simulink model "pitch_loop"  (Simulink 8.2)
settings: Solver=ode45  StartTime=0.0  StopTime=500  FixedStep=0.01  RelTol=1e-3
undefined symbols (not defined in the file): P
settings Model: Creator=paul  LastModifiedBy=paul
settings DataIOCC: SignalLoggingSaveFormat=Dataset
settings OptimizationCC: ExpressionDepthLimit=128
settings DebuggingCC: FcnCallInpInsideContextMsg=EnableAllAsError  StateNameClashWarn=none
settings GRTTargetCC: CombineOutputUpdateFcns=on  GRTInterface=off

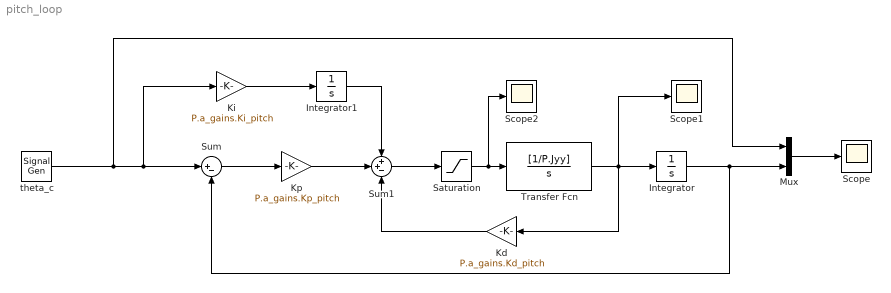
== system pitch_loop ==
  Integrator : Integrator
  Integrator1 : Integrator
  Kd : Gain  Gain=P.a_gains.Kd_pitch
  Ki : Gain  Gain=P.a_gains.Ki_pitch
  Kp : Gain  Gain=P.a_gains.Kp_pitch
  Mux : Mux  Inputs=2
  Saturation : Saturate  UpperLimit=P.T_theta_max  LowerLimit=-P.T_theta_max
  Scope : Scope
  Scope1 : Scope
  Scope2 : Scope
      settings: SaveName=ScopeData2
  Sum : Sum  Inputs=|+-
  Sum1 : Sum  Inputs=++-
  Transfer Fcn : TransferFcn  Numerator=[1/P.Jyy]  Denominator=[1 0]
  theta_c : SignalGenerator  WaveForm=square  Amplitude=0.25  Frequency=0.05
  wires:
  Integrator1/1 -> Sum1/1
  Ki/1 -> Integrator1/1
  Sum/1 -> Kp/1
  Kp/1 -> Sum1/2
  Sum1/1 -> Saturation/1
  Saturation/1 -> Scope2/1, Transfer Fcn/1
  Mux/1 -> Scope/1
  theta_c/1 -> Mux/1, Ki/1, Sum/1
  Kd/1 -> Sum1/3
  Transfer Fcn/1 -> Scope1/1, Kd/1, Integrator/1
  Integrator/1 -> Sum/2, Mux/2
